simulink model "FullCar_BodyModel"  (R2018b)
settings: Solver=VariableStepAuto  StartTime=0.0  StopTime=10.0  RelTol=1e-3
values from neighbouring files (symbols this model uses):
  a = 1.25    [SetCoefficients.m]
  b = 1.4    [SetCoefficients.m]
  g = 9.81    [SetCoefficients.m]
  I_phi = 1000    [SetCoefficients.m]
  I_theta = 600    [SetCoefficients.m]
  mb = 1000    [SetCoefficients.m]
  s = 3    [SetCoefficients.m]
settings Model: Creator=joebe  LastModifiedBy=joebe

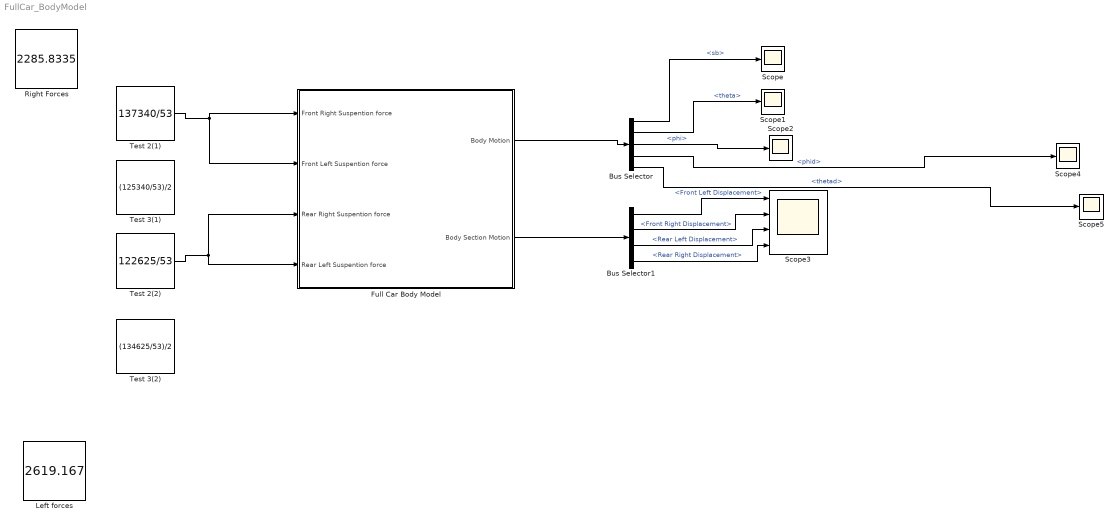
== system FullCar_BodyModel ==
  Bus Selector : BusSelector  OutputSignals=Body Vertical Motion.sb,body pitch motion.theta,Body Pitch motion.phi,Body Pitch motion.phid,body pitch motion.thetad
  Bus Selector1 : BusSelector  OutputSignals=Front Left Body Motion.Front Left Displacement,Front Right Body Motion.Front Right Displacement,Rear Left Body Motion.Rear Left Displacement,Rear Right Body Motion.Rear Right Displacement
  Full Car Body Model : Subsystem
  Left forces : Constant  Value=2619.167
  Right Forces : Constant  Value=2285.8335
  Scope{,1..2,4..5} (5 alike) : Scope
  Scope3 : Scope  NumInputPorts=4
  Test 2(1) : Constant  Value=137340/53
  Test 2(2) : Constant  Value=122625/53
  Test 3(1) : Constant  Value=(125340/53)/2
  Test 3(2) : Constant  Value=(134625/53)/2
  wires:
  Full Car Body Model/1(Body Motion) -> Bus Selector/1
  Bus Selector/3 -> Scope2/1  "<phi>"
  Bus Selector/2 -> Scope1/1  "<theta>"
  Bus Selector/1 -> Scope/1  "<sb>"
  Full Car Body Model/2(Body Section Motion) -> Bus Selector1/1
  Bus Selector1/1 -> Scope3/1  "<Front Left Displacement>"
  Bus Selector1/2 -> Scope3/2  "<Front Right Displacement>"
  Bus Selector1/3 -> Scope3/3  "<Rear Left Displacement>"
  Bus Selector1/4 -> Scope3/4  "<Rear Right Displacement>"
  Test 2(2)/1 -> Full Car Body Model/4(Rear Left Suspention force), Full Car Body Model/3(Rear Right Suspention force)
  Test 2(1)/1 -> Full Car Body Model/1(Front Right Suspention force), Full Car Body Model/2(Front Left Suspention force)
  Bus Selector/4 -> Scope4/1  "<phid>"
  Bus Selector/5 -> Scope5/1  "<thetad>"

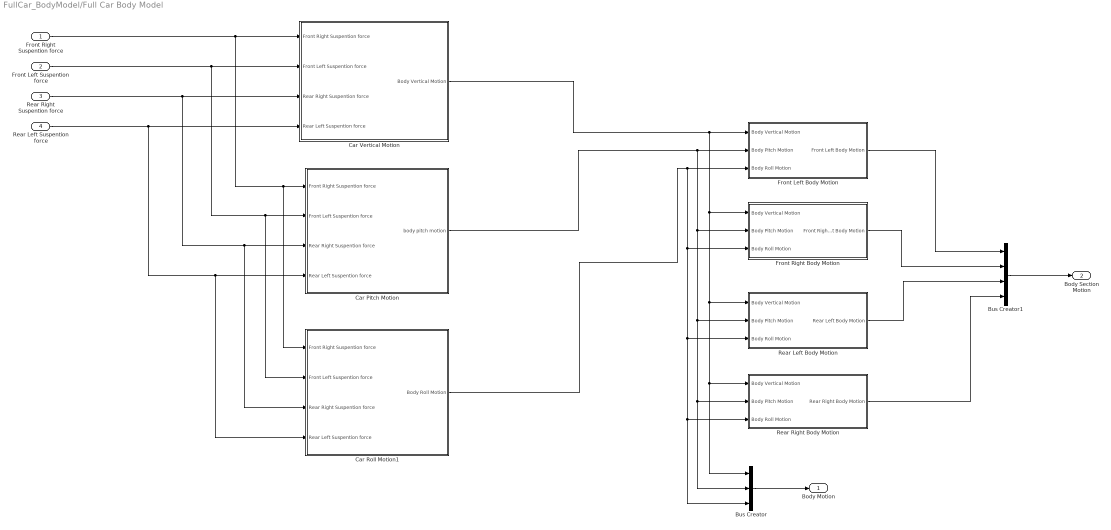
== system FullCar_BodyModel/Full Car Body Model ==
  Front Right Suspention force : Inport
  Front Left Suspention force : Inport  Port=2
  Rear Right Suspention force : Inport  Port=3
  Rear Left Suspention force : Inport  Port=4
  Bus Creator : BusCreator  Inputs=3
  Bus Creator1 : BusCreator  Inputs=4
  Car Pitch Motion : Subsystem
  Car Roll Motion1 : Subsystem
  Car Vertical Motion : Subsystem
  Front Left Body Motion : Subsystem
  "Front Right Body Motion " : Subsystem
  Rear Left Body Motion : Subsystem
  Rear Right Body Motion : Subsystem
  Body Motion : Outport
  Body Section Motion : Outport  Port=2
  wires:
  Front Right Suspention force/1 -> Car Roll Motion1/1(Front Right Suspention force), Car Pitch Motion/1(Front Right Suspention force), Car Vertical Motion/1(Front Right Suspention force)
  Front Left Suspention force/1 -> Car Roll Motion1/2(Front Left Suspention force), Car Pitch Motion/2(Front Left Suspention force), Car Vertical Motion/2(Front Left Suspention force)
  Rear Right Suspention force/1 -> Car Roll Motion1/3(Rear Right Suspention force), Car Pitch Motion/3(Rear Right Suspention force), Car Vertical Motion/3(Rear Right Suspention force)
  Car Vertical Motion/1(Body Vertical Motion) -> Bus Creator/1, Rear Right Body Motion/1(Body Vertical Motion), Rear Left Body Motion/1(Body Vertical Motion), "Front Right Body Motion "/1(Body Vertical Motion), Front Left Body Motion/1(Body Vertical Motion)
  Rear Left Suspention force/1 -> Car Roll Motion1/4(Rear Left Suspention force), Car Pitch Motion/4(Rear Left Suspention force), Car Vertical Motion/4(Rear Left Suspention force)
  Car Roll Motion1/1(Body Roll Motion) -> Bus Creator/3, Rear Right Body Motion/3(Body Roll Motion), Rear Left Body Motion/3(Body Roll Motion), "Front Right Body Motion "/3(Body Roll Motion), Front Left Body Motion/3(Body Roll Motion)
  Car Pitch Motion/1(body pitch motion) -> Bus Creator/2, Rear Right Body Motion/2(Body Pitch Motion), Rear Left Body Motion/2(Body Pitch Motion), "Front Right Body Motion "/2(Body Pitch Motion), Front Left Body Motion/2(Body Pitch Motion)
  Bus Creator/1 -> Body Motion/1
  Bus Creator1/1 -> Body Section Motion/1
  Front Left Body Motion/1(Front Left Body Motion) -> Bus Creator1/1
  "Front Right Body Motion "/1(Front Right Body Motion) -> Bus Creator1/2
  Rear Left Body Motion/1(Rear Left Body Motion) -> Bus Creator1/3
  Rear Right Body Motion/1(Rear Right Body Motion) -> Bus Creator1/4

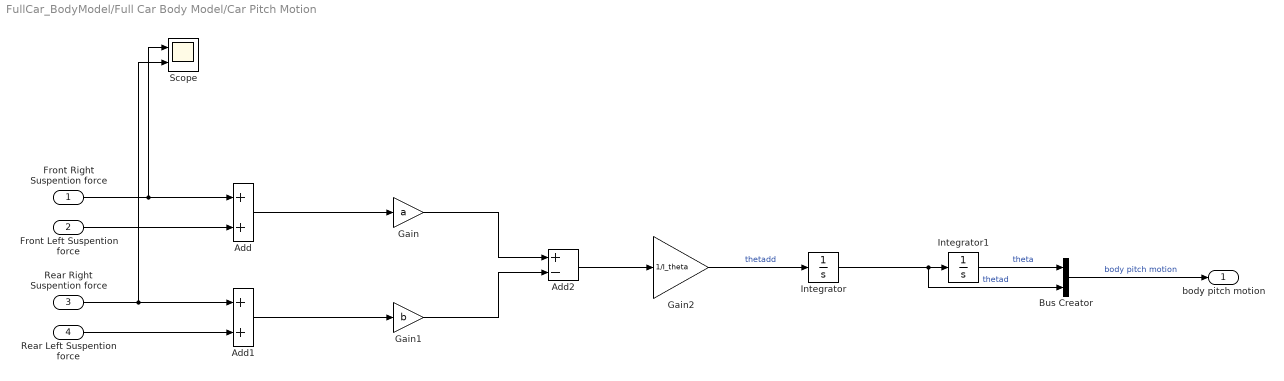
== system FullCar_BodyModel/Full Car Body Model/Car Pitch Motion ==
  Front Right Suspention force : Inport
  Front Left Suspention force : Inport  Port=2
  Rear Right Suspention force : Inport  Port=3
  Rear Left Suspention force : Inport  Port=4
  Add : Sum
  Add1 : Sum
  Add2 : Sum  Inputs=+-
  Bus Creator : BusCreator  Inputs=2
  Gain : Gain  Gain=a
  Gain1 : Gain  Gain=b
  Gain2 : Gain  Gain=1/I_theta
  Integrator : Integrator
  Integrator1 : Integrator
  Scope : Scope  NumInputPorts=2
  body pitch motion : Outport
  wires:
  Gain/1 -> Add2/1
  Gain1/1 -> Add2/2
  Gain2/1 -> Integrator/1  "thetadd"
  Add1/1 -> Gain1/1
  Add2/1 -> Gain2/1
  Integrator/1 -> Bus Creator/2, Integrator1/1  "thetad"
  Rear Right Suspention force/1 -> Add1/1, Scope/2
  Add/1 -> Gain/1
  Integrator1/1 -> Bus Creator/1  "theta"
  Front Right Suspention force/1 -> Scope/1, Add/1
  Bus Creator/1 -> body pitch motion/1  "body pitch motion"
  Front Left Suspention force/1 -> Add/2
  Rear Left Suspention force/1 -> Add1/2

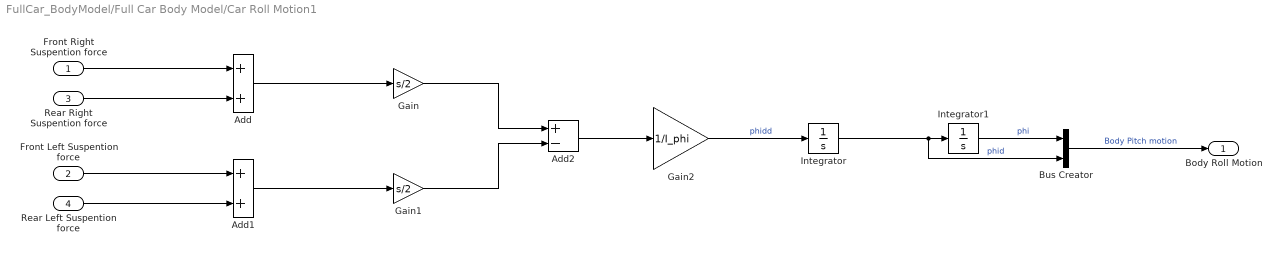
== system FullCar_BodyModel/Full Car Body Model/Car Roll Motion1 ==
  Front Right Suspention force : Inport
  Front Left Suspention force : Inport  Port=2
  Rear Right Suspention force : Inport  Port=3
  Rear Left Suspention force : Inport  Port=4
  Add : Sum
  Add1 : Sum
  Add2 : Sum  Inputs=+-
  Bus Creator : BusCreator  Inputs=2
  Gain : Gain  Gain=s/2
  Gain1 : Gain  Gain=s/2
  Gain2 : Gain  Gain=1/I_phi
  Integrator : Integrator
  Integrator1 : Integrator
  Body Roll Motion : Outport
  wires:
  Gain/1 -> Add2/1
  Gain1/1 -> Add2/2
  Gain2/1 -> Integrator/1  "phidd"
  Add1/1 -> Gain1/1
  Add2/1 -> Gain2/1
  Integrator/1 -> Bus Creator/2, Integrator1/1  "phid"
  Add/1 -> Gain/1
  Integrator1/1 -> Bus Creator/1  "phi"
  Front Right Suspention force/1 -> Add/1
  Bus Creator/1 -> Body Roll Motion/1  "Body Pitch motion"
  Rear Left Suspention force/1 -> Add1/2
  Rear Right Suspention force/1 -> Add/2
  Front Left Suspention force/1 -> Add1/1

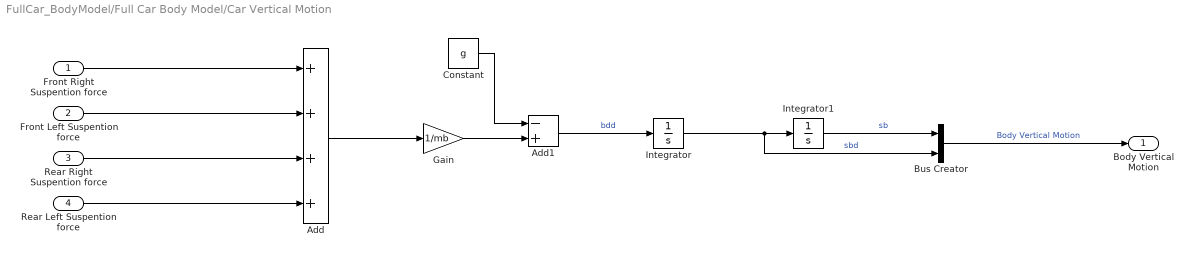
== system FullCar_BodyModel/Full Car Body Model/Car Vertical Motion ==
  Front Right Suspention force : Inport
  Front Left Suspention force : Inport  Port=2
  Rear Right Suspention force : Inport  Port=3
  Rear Left Suspention force : Inport  Port=4
  Add : Sum  Inputs=4
  Add1 : Sum  Inputs=-+
  Bus Creator : BusCreator  Inputs=2
  Constant : Constant  Value=g
  Gain : Gain  Gain=1/mb
  Integrator : Integrator
  Integrator1 : Integrator
  Body Vertical Motion : Outport
  wires:
  Constant/1 -> Add1/1
  Add1/1 -> Integrator/1  "bdd"
  Add/1 -> Gain/1
  Integrator/1 -> Bus Creator/2, Integrator1/1  "sbd"
  Integrator1/1 -> Bus Creator/1  "sb"
  Rear Right Suspention force/1 -> Add/3
  Gain/1 -> Add1/2
  Bus Creator/1 -> Body Vertical Motion/1  "Body Vertical Motion"
  Front Left Suspention force/1 -> Add/2
  Front Right Suspention force/1 -> Add/1
  Rear Left Suspention force/1 -> Add/4

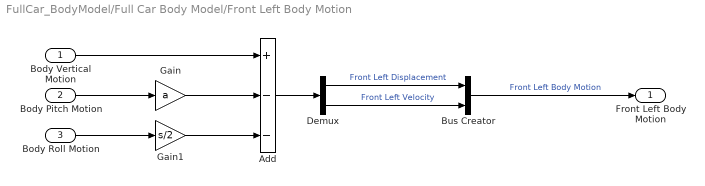
== system FullCar_BodyModel/Full Car Body Model/Front Left Body Motion ==
  Body Vertical Motion : Inport
  Body Pitch Motion : Inport  Port=2
  Body Roll Motion : Inport  Port=3
  Add : Sum  Inputs=+--
  Bus Creator : BusCreator  Inputs=2
  Demux : Demux  Outputs=2
  Gain : Gain  Gain=a
  Gain1 : Gain  Gain=s/2
  Front Left Body Motion : Outport
  wires:
  Body Roll Motion/1 -> Gain1/1
  Gain1/1 -> Add/3
  Body Pitch Motion/1 -> Gain/1
  Gain/1 -> Add/2
  Body Vertical Motion/1 -> Add/1
  Add/1 -> Demux/1
  Demux/1 -> Bus Creator/1  "Front Left Displacement"
  Demux/2 -> Bus Creator/2  "Front Left Velocity"
  Bus Creator/1 -> Front Left Body Motion/1  "Front Left Body Motion"

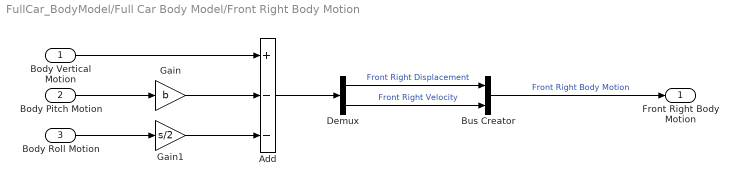
== system FullCar_BodyModel/Full Car Body Model/Front Right Body Motion  ==
  Body Vertical Motion : Inport
  Body Pitch Motion : Inport  Port=2
  Body Roll Motion : Inport  Port=3
  Add : Sum  Inputs=+--
  Bus Creator : BusCreator  Inputs=2
  Demux : Demux  Outputs=2
  Gain : Gain  Gain=b
  Gain1 : Gain  Gain=s/2
  Front Right Body Motion : Outport
  wires:
  Body Roll Motion/1 -> Gain1/1
  Gain1/1 -> Add/3
  Body Pitch Motion/1 -> Gain/1
  Gain/1 -> Add/2
  Body Vertical Motion/1 -> Add/1
  Demux/1 -> Bus Creator/1  "Front Right Displacement"
  Demux/2 -> Bus Creator/2  "Front Right Velocity"
  Add/1 -> Demux/1
  Bus Creator/1 -> Front Right Body Motion/1  "Front Right Body Motion"

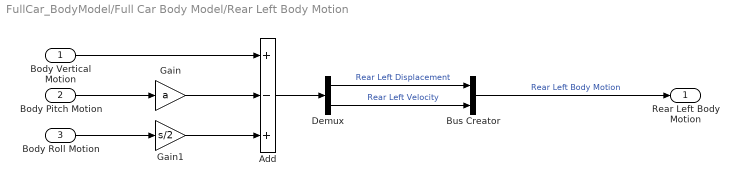
== system FullCar_BodyModel/Full Car Body Model/Rear Left Body Motion ==
  Body Vertical Motion : Inport
  Body Pitch Motion : Inport  Port=2
  Body Roll Motion : Inport  Port=3
  Add : Sum  Inputs=+-+
  Bus Creator : BusCreator  Inputs=2
  Demux : Demux  Outputs=2
  Gain : Gain  Gain=a
  Gain1 : Gain  Gain=s/2
  Rear Left Body Motion : Outport
  wires:
  Body Roll Motion/1 -> Gain1/1
  Gain1/1 -> Add/3
  Body Pitch Motion/1 -> Gain/1
  Gain/1 -> Add/2
  Body Vertical Motion/1 -> Add/1
  Demux/1 -> Bus Creator/1  "Rear Left Displacement"
  Demux/2 -> Bus Creator/2  "Rear Left Velocity"
  Add/1 -> Demux/1
  Bus Creator/1 -> Rear Left Body Motion/1  "Rear Left Body Motion"

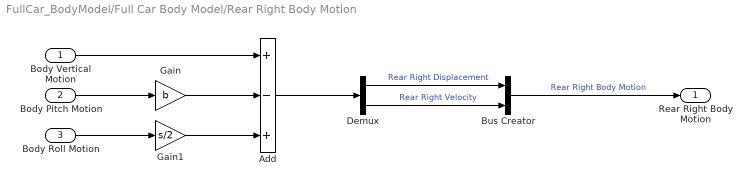
== system FullCar_BodyModel/Full Car Body Model/Rear Right Body Motion ==
  Body Vertical Motion : Inport
  Body Pitch Motion : Inport  Port=2
  Body Roll Motion : Inport  Port=3
  Add : Sum  Inputs=+-+
  Bus Creator : BusCreator  Inputs=2
  Demux : Demux  Outputs=2
  Gain : Gain  Gain=b
  Gain1 : Gain  Gain=s/2
  Rear Right Body Motion : Outport
  wires:
  Body Roll Motion/1 -> Gain1/1
  Gain1/1 -> Add/3
  Body Pitch Motion/1 -> Gain/1
  Gain/1 -> Add/2
  Body Vertical Motion/1 -> Add/1
  Demux/1 -> Bus Creator/1  "Rear Right Displacement"
  Demux/2 -> Bus Creator/2  "Rear Right Velocity"
  Add/1 -> Demux/1
  Bus Creator/1 -> Rear Right Body Motion/1  "Rear Right Body Motion"
